simulink model "Lab_3_Velocity_Controlled_Landing_Module"  (R2019b)
settings: Solver=VariableStepAuto  StartTime=0.0  StopTime=10.0  RelTol=1e-3
libraries: simulink x1
settings Model: DataDictionary=Lab_3_Common_Data.sldd  EnableAccessToBaseWorkspace=off  Creator=rollends  LastModifiedBy=Arjun
settings DebuggingCC: ArithmeticOperatorsInVariantConditions=warning
settings SFSimCC: CustomCodeUndefinedFunction=UseInterfaceOnly

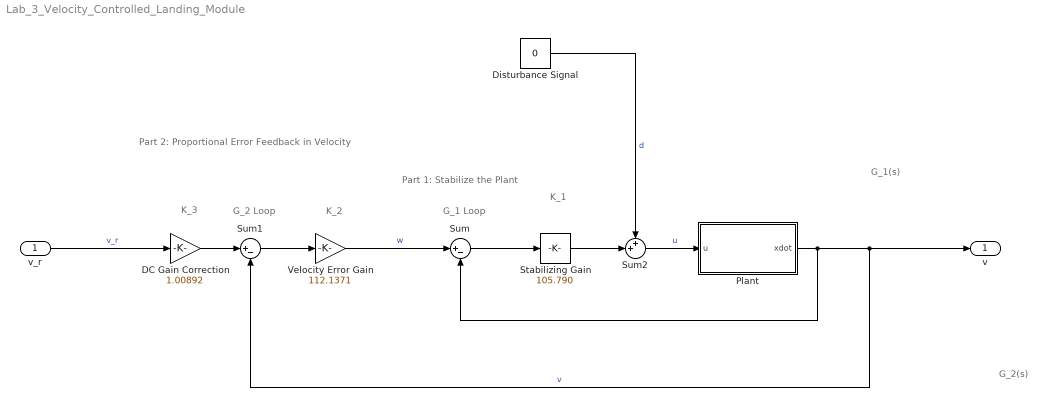
== system Lab_3_Velocity_Controlled_Landing_Module ==
  note: K_3
  note: G_2 Loop
  note: K_2
  note: K_1
  note: G_1 Loop
  note: Part 2: Proportional Error Feedback in Velocity
  note: Part 1: Stabilize the Plant
  note: G_1(s)
  note: G_2(s)
  v_r : Inport
  DC Gain Correction : Gain  Gain=1.00892
  Disturbance Signal : Constant  Value=0  OutDataTypeStr=Inherit: Inherit via back propagation
  "Plant " : Subsystem
  Stabilizing Gain : simulink/Math Operations/Slider Gain  gain=105.790  low=1  high=500
  Sum : Sum  Inputs=|+-
  Sum1 : Sum  Inputs=|+-
  Sum2 : Sum  Inputs=++|
  Velocity Error Gain : Gain  Gain=112.1371
  v : Outport
  wires:
  v_r/1 -> DC Gain Correction/1  "v_r"
  DC Gain Correction/1 -> Sum1/1
  Velocity Error Gain/1 -> Sum/1  "w"
  "Plant "/1(xdot) -> Sum/2, Sum1/2, v/1  "v"
  Sum/1 -> Stabilizing Gain/1
  Sum1/1 -> Velocity Error Gain/1
  Sum2/1 -> "Plant "/1(u)  "u"
  Disturbance Signal/1 -> Sum2/1  "d"
  Stabilizing Gain/1 -> Sum2/2

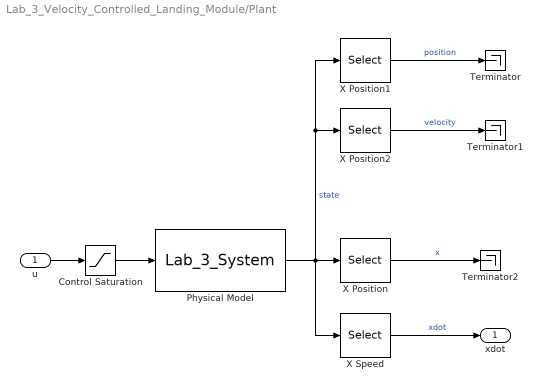
== system Lab_3_Velocity_Controlled_Landing_Module/Plant  ==
  u : Inport
  Control Saturation : Saturate  UpperLimit=10000  LowerLimit=-10000
  Physical Model : M-S-Function  FunctionName=Lab_3_System  Parameters=InitialCondition
  Terminator : Terminator
  Terminator1 : Terminator
  Terminator2 : Terminator
  X Position : Selector  InputPortWidth=4  IndexOptions=Index vector (dialog)  Indices=[1]  OutputSizes=1
  X Position1 : Selector  InputPortWidth=4  IndexOptions=Index vector (dialog)  Indices=[1 2]  OutputSizes=1
  X Position2 : Selector  InputPortWidth=4  IndexOptions=Index vector (dialog)  Indices=[3 4]  OutputSizes=1
  X Speed : Selector  InputPortWidth=4  IndexOptions=Index vector (dialog)  Indices=[3]  OutputSizes=1
  xdot : Outport
  wires:
  X Position/1 -> Terminator2/1  "x"
  u/1 -> Control Saturation/1
  Control Saturation/1 -> Physical Model/1
  X Speed/1 -> xdot/1  "xdot"
  Physical Model/1 -> X Position2/1, X Position1/1, X Speed/1, X Position/1  "state"
  X Position1/1 -> Terminator/1  "position"
  X Position2/1 -> Terminator1/1  "velocity"
